simulink library "tetherInternalForces_ul"  (R2018b)
settings: Solver=VariableStepAuto  StartTime=0.0  StopTime=10.0  RelTol=1e-3
values from neighbouring files (symbols this model uses):
  dia_t = 0.01    [tetherInternalForces_ts.m]
  E = 3.8e9    (= 3800000000)    [tetherInternalForces_ts.m]
  mass = 100    [tetherInternalForces_ts.m]
  N = 2    [tetherInternalForces_ts.m]
  zeta = 0.05    [tetherInternalForces_ts.m]
settings Model: Creator=asiddiq2  LastModifiedBy=asiddiq2

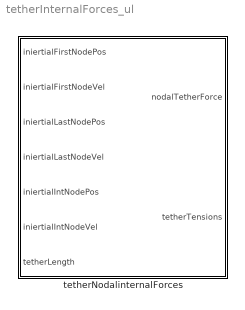
== system tetherInternalForces_ul ==
  tetherNodalinternalForces : Subsystem  mask{massBdy=mass, numNode=N, thrDia=dia_t, thrYoungs=E, thrZeta=zeta}
      mask prompts: massBdy "Vehicle Mass (kg)"; numNode "Number of nodes"; thrDia "Tether diameter"; thrYoungs "Youngs Modulus"; thrZeta "Damping ratio"
      mask DialogControl Container3 Prompt: Vehicle

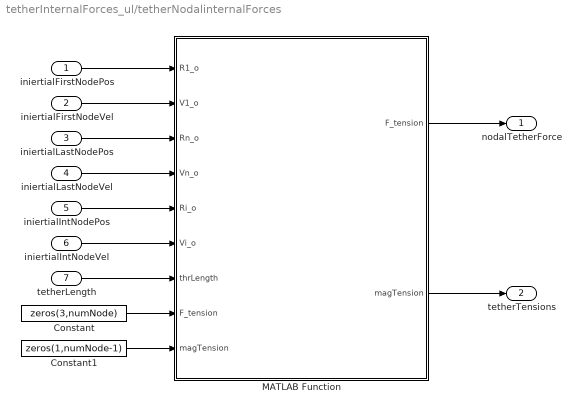
== system tetherInternalForces_ul/tetherNodalinternalForces ==
  iniertialFirstNodePos : Inport
  iniertialFirstNodeVel : Inport  Port=2
  iniertialLastNodePos : Inport  Port=3
  iniertialLastNodeVel : Inport  Port=4
  iniertialIntNodePos : Inport  Port=5
  iniertialIntNodeVel : Inport  Port=6
  tetherLength : Inport  Port=7
  Constant : Constant  Value=zeros(3,numNode)  VectorParams1D=off
  Constant1 : Constant  Value=zeros(1,numNode-1)  VectorParams1D=off
  MATLAB Function : MATLAB Function  TreatAsAtomicUnit=on
  nodalTetherForce : Outport
  tetherTensions : Outport  Port=2
  wires:
  MATLAB Function/2(magTension) -> tetherTensions/1
  iniertialLastNodePos/1 -> MATLAB Function/3(Rn_o)
  iniertialLastNodeVel/1 -> MATLAB Function/4(Vn_o)
  iniertialIntNodePos/1 -> MATLAB Function/5(Ri_o)
  iniertialIntNodeVel/1 -> MATLAB Function/6(Vi_o)
  iniertialFirstNodePos/1 -> MATLAB Function/1(R1_o)
  iniertialFirstNodeVel/1 -> MATLAB Function/2(V1_o)
  tetherLength/1 -> MATLAB Function/7(thrLength)
  Constant/1 -> MATLAB Function/8("F_tension ")
  Constant1/1 -> MATLAB Function/9("magTension ")
  MATLAB Function/1(F_tension) -> nodalTetherForce/1

== matlab function tetherInternalForces_ul/tetherNodalinternalForces/MATLAB Function ==
  data: R1_o input; V1_o input; Rn_o input; Vn_o input; F_tension output; Ri_o input; Vi_o input; thrLength input; F_tension input; magTension input; numNode parameter; massBdy parameter; thrZeta parameter; thrYoungs parameter; magTension output; thrDia parameter
function [F_tension,magTension]  = fcn(R1_o,V1_o,Rn_o,Vn_o,Ri_o,Vi_o,thrLength,F_tension,magTension,...
    numNode, massBdy, thrZeta, thrYoungs, thrDia)

if numNode == 2
    Ri_o = [R1_o Rn_o];
    Vi_o = [V1_o Vn_o];
else
    Ri_o = [R1_o Ri_o Rn_o];
    Vi_o = [V1_o Vi_o Vn_o];
end

% cross sectional area
CS = (pi/4)*thrDia^2;

% total spring stiffness
k_tot = thrYoungs*CS/thrLength;

% total damping coefficient
c_tot = thrZeta*2*sqrt(k_tot*massBdy);

% inidividual spring stiffness and damping
kElem = k_tot*(numNode-1);
cElem = c_tot*(numNode-1);
LiElem = thrLength/(numNode-1);

% determine distance between nodes and the derivatives of each element
di = zeros(numNode-1,1);
direction = zeros(3,numNode-1);
di_dot = zeros(numNode-1,1);
Tk = zeros(numNode-1,1);
Td = zeros(numNode-1,1);
F_t_i = zeros(3,numNode-1);


for ii = 1:numNode-1
    di(ii) = norm(Ri_o(:,ii+1) - Ri_o(:,ii));
    direction(:,ii) = (Ri_o(:,ii+1) - Ri_o(:,ii))/di(ii);
    di_dot(ii) = dot((Ri_o(:,ii+1) - Ri_o(:,ii)),(Vi_o(:,ii+1) - Vi_o(:,ii)))/di(ii);
    
end

% spring and damper forces
for ii = 1:numNode-1
    if di(ii) > LiElem
        Tk(ii) = kElem*(di(ii) - LiElem);
        Td(ii) = cElem*di_dot(ii);
        F_t_i(:,ii) = (Tk(ii) + Td(ii))*direction(:,ii);
        magTension(ii) = norm(F_t_i(:,ii));
    else
        Tk(ii) = 0;
        Td(ii) = 0;
        F_t_i(:,ii) = (Tk(ii) + Td(ii))*direction(:,ii);
        magTension(ii) = norm(F_t_i(:,ii));
        
    end
end

for ii = 1:numNode
    if ii == 1
        F_tension(:,ii) = F_t_i(:,ii);
    elseif ii > 1 && ii < numNode
        F_tension(:,ii) = F_t_i(:,ii) - F_t_i(:,ii-1);
    elseif ii == numNode
        F_tension(:,ii) = -F_t_i(:,ii-1);
    end
end


end
